simulink model "BMS_Submodel"  (R2026a)
settings: Solver=FixedStepAuto  StopTime=3600  FixedStep=0.01
values from neighbouring files (symbols this model uses):
  a_montes = 0.869    [WS_Variables.mat]
  alpha_cal = 0.384    [WS_Variables.mat]
  dt_h = 1    [WS_Variables.mat]    (also in validate_fixes.m)
  Ea_cal = 20592    [WS_Variables.mat]
  F_const = 96485    [WS_Variables.mat]
  I_ch_max = 3    [WS_Variables.mat]
  I_dis_max = 3    [WS_Variables.mat]
  k0_cal = 0.142    [WS_Variables.mat]
  kcal_ref = 0.0003694    [WS_Variables.mat]
  kCch = 0.1038    [WS_Variables.mat]
  kCdch = 0.296    [WS_Variables.mat]
  kcyc = 0.003414    [WS_Variables.mat]
  kDODc = 0.0046    [WS_Variables.mat]
  kmSOC = 0.0513    [WS_Variables.mat]
  kT = 5.8755    [WS_Variables.mat]
  mSOCref = 0.42    [WS_Variables.mat]
  Q_nom = 3    [WS_Variables.mat]
  R_ch_2D = [0.0536 0.0408 0.0368 0.0344 0.0288 0.0264 0.024 0.0595555555556 0.0453333333333 0.0408888888889 0.0382222222222 0.032 ... (77 elements, 7x11)]    [WS_Variables.mat]
  R_dis_2D = [0.1152 0.088 0.0768 0.072 0.064 0.0576 0.0528 0.0936 0.0715 0.0624 0.0585 0.052 ... (77 elements, 7x11)]    [WS_Variables.mat]
  R_gas = 8.314462618    [WS_Variables.mat]
  SOC0 = 0.5    [WS_Variables.mat]
  SOC_grid = [0 0.1 0.2 0.3 0.4 0.5 0.6 0.7 0.8 0.9 1]    [WS_Variables.mat]
  SOC_max = 0.95    [WS_Variables.mat]
  SOC_min = 0.05    [WS_Variables.mat]
  T_degC = 25    [WS_Variables.mat]
  T_grid_C = [10 20 25 30 40 50 60]    [WS_Variables.mat]
  Tref_cal = 298.15    [WS_Variables.mat]
  Tref_K = 298    [WS_Variables.mat]
  Ua_ref = 0.123    [WS_Variables.mat]
  V_nom = 3.2    [WS_Variables.mat]
undefined symbols (not defined in the file or in its folder): b_I, b_T, b_V, DiscIntNeverNeededParam, g_I, GridSearch_EN, I_cmd, nseedI, nseedT, nseedV, SOC0_est, SOH_Grid, step_size
libraries: simulink x5, sl_discontinuities x1
settings Model: Creator=diaag  LastModifiedBy=diaag

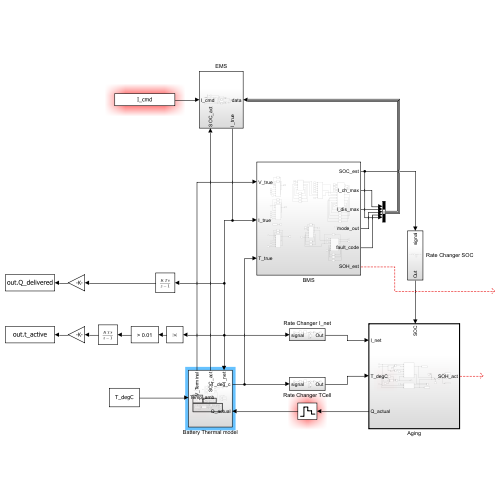
[thumbnail: Simulink's stored preview of the top-level diagram]
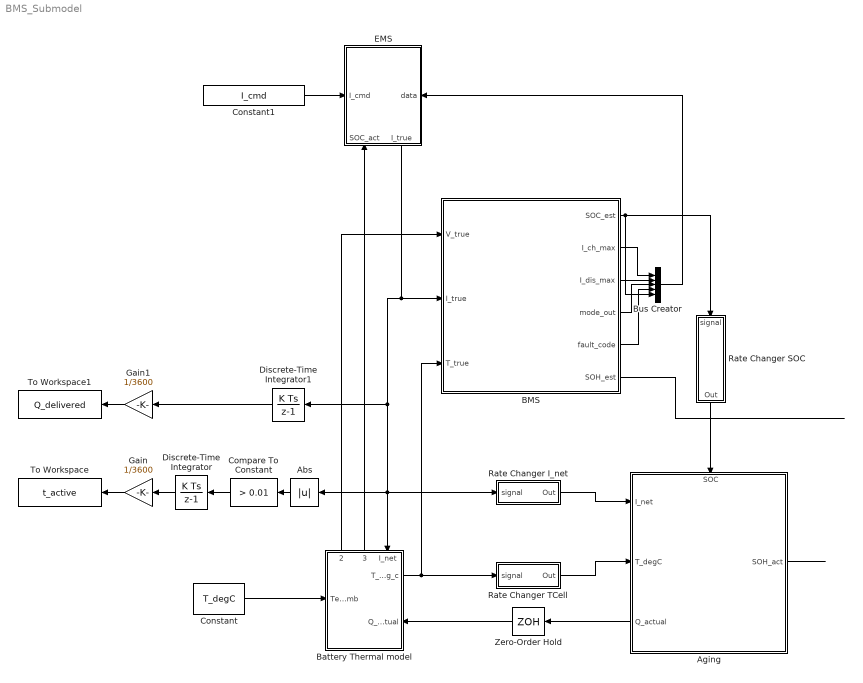
== system BMS_Submodel ==
  Abs : Abs  SaturateOnIntegerOverflow=off
  Aging : Subsystem  TreatAsAtomicUnit=on  SystemSampleTime=3600
      settings: PortSchema="{\"entries\":[{\"content\":{\"sides\":[{\"content\":{\"connectorIds\":[\"In1\",\"In2\",\"Out2\"]},\"type\":\"ConnectorPlacement.EquallySpacedRectSide\",\"uuid\":\"e6db651b-c6dd-4cac-b472-a1afbe19ba44\"},{\"content\":{\"connectorIds\":[\"Out1\"],\"side\":\"RIGHT\"},\"type\":\"ConnectorPlacement.EquallySpacedRectSide\",\"uuid\":\"7d47abdb-bdb7-40fd-84ce-b87800cb59fa\"},{\"content\":{\"connectorIds\":[\"In3\"],\"side\":\"TOP\"},\"type\":\"ConnectorPlacement.EquallySpacedRectSide\",\"uuid\":\"eff55775-1cf2-424a-af47-d3042302cf74\"}]},\"type\":\"ConnectorPlacement.EquallySpacedConnector\",\"uuid\":\"45aa8090-c1c1-4510-ac4d-5e24907f6a7b\"}],\"packageUris\":[\"http://schema.mathworks.com/mf0/Connector/R2020b\"],\"version\":\"1.0\"}"
  BMS : Subsystem
  Battery Thermal model : Subsystem
      settings: PortSchema="{\"entries\":[{\"content\":{\"sides\":[{\"content\":{\"connectorIds\":[\"Out2\",\"Out3\",\"In1\"]},\"type\":\"ConnectorPlacement.EquallySpacedRectSide\",\"uuid\":\"e701b896-6e4d-4329-a4c3-4a880497ce66\"},{\"content\":{\"side\":\"RIGHT\"},\"type\":\"ConnectorPlacement.EquallySpacedRectSide\",\"uuid\":\"c3e4b798-963d-4ee1-99ed-454cd6d82987\"},{\"content\":{\"connectorIds\":[\"In2\"],\"side\":\"TOP\"},\"type\":\"ConnectorPlacement.EquallySpacedRectSide\",\"uuid\":\"33ef008e-5290-4140-baf3-69d32b77873e\"},{\"content\":{\"connectorIds\":[\"Out1\",\"In3\"],\"side\":\"BOTTOM\"},\"type\":\"ConnectorPlacement.EquallySpacedRectSide\",\"uuid\":\"032c09d0-f76a-4e61-be97-2904950a15a3\"}]},\"type\":\"ConnectorPlacement.EquallySpacedConnector\",\"uuid\":\"523c5e39-84aa-4d7a-8c26-e0b756ae59f3\"}],\"packageUris\":[\"http://schema.mathworks.com/mf0/Connector/R2020b\"],\"version\":\"1.0\"}"
  Bus Creator : BusCreator  Inputs=5
  Compare To Constant : simulink/Logic and Bit Operations/Compare To Constant  relop=>  const=0.01  OutDataTypeStr=boolean
  Constant : Constant  Value=T_degC
  Constant1 : Constant  Value=I_cmd
  Discrete-Time Integrator : DiscreteIntegrator  SampleTime=-1  OutDataTypeStr=double  ICPrevOutput=DiscIntNeverNeededParam  ICPrevScaledInput=DiscIntNeverNeededParam
  Discrete-Time Integrator1 : DiscreteIntegrator  SampleTime=-1  ICPrevOutput=DiscIntNeverNeededParam  ICPrevScaledInput=DiscIntNeverNeededParam
  EMS : Subsystem
      settings: PortSchema="{\"entries\":[{\"content\":{\"sides\":[{\"content\":{\"connectorIds\":[\"In1\"]},\"type\":\"ConnectorPlacement.EquallySpacedRectSide\",\"uuid\":\"d23f0ade-e6c5-473f-be03-48db0421b0ac\"},{\"content\":{\"connectorIds\":[\"In3\"],\"side\":\"RIGHT\"},\"type\":\"ConnectorPlacement.EquallySpacedRectSide\",\"uuid\":\"35749c49-4500-4b94-810c-884c3143aa7f\"},{\"content\":{\"side\":\"TOP\"},\"type\":\"ConnectorPlacement.EquallySpacedRectSide\",\"uuid\":\"e0e4976e-0f30-4d6f-9552-049331019e02\"},{\"content\":{\"connectorIds\":[\"In2\",\"Out1\"],\"side\":\"BOTTOM\"},\"type\":\"ConnectorPlacement.EquallySpacedRectSide\",\"uuid\":\"1cb18c9d-5935-496e-9b55-fe9d42ae6b73\"}]},\"type\":\"ConnectorPlacement.EquallySpacedConnector\",\"uuid\":\"12474735-7fad-4afe-9583-bac38bcbc472\"}],\"packageUris\":[\"http://schema.mathworks.com/mf0/Connector/R2020b\"],\"version\":\"1.0\"}"
  Gain : Gain  Gain=1/3600  OutDataTypeStr=double
  Gain1 : Gain  Gain=1/3600  OutDataTypeStr=double
  Rate Changer I_net : Subsystem
  Rate Changer SOC : Subsystem
  Rate Changer TCell : Subsystem
  To Workspace : ToWorkspace  VariableName=t_active  SaveFormat=Timeseries  SampleTime=-1
      settings: MaxDataPoints=1
  To Workspace1 : ToWorkspace  VariableName=Q_delivered  SaveFormat=Timeseries  SampleTime=-1
      settings: MaxDataPoints=1
  Zero-Order Hold : ZeroOrderHold  SampleTime=3600/step_size
  wires:
  Rate Changer I_net/1(Out) -> Aging/1(I_net)
  Rate Changer SOC/1(Out) -> Aging/3(SOC)
  Rate Changer TCell/1(Out) -> Aging/2(T_degC)
  Zero-Order Hold/1 -> Battery Thermal model/3(Q_actual)
  Aging/2(Q_actual) -> Zero-Order Hold/1
  Battery Thermal model/1(T_deg_c) -> BMS/3(T_true), Rate Changer TCell/1(signal)
  Battery Thermal model/2(V_Terminal) -> BMS/1(V_true)
  EMS/1(I_true) -> Discrete-Time Integrator1/1, Abs/1, Rate Changer I_net/1(signal), Battery Thermal model/1(I_net), BMS/2(I_true)
  BMS/1(SOC_est) -> Rate Changer SOC/1(signal), Bus Creator/5
  BMS/6(SOH_est) -> ?
  Aging/1(SOH_act) -> ?
  BMS/2(I_ch_max) -> Bus Creator/1
  BMS/3(I_dis_max) -> Bus Creator/2
  BMS/4(mode_out) -> Bus Creator/3
  BMS/5(fault_code) -> Bus Creator/4
  Bus Creator/1 -> EMS/3(data)
  Constant/1 -> Battery Thermal model/2(Temp_amb)
  Constant1/1 -> EMS/1(I_cmd)
  Abs/1 -> Compare To Constant/1
  Compare To Constant/1 -> Discrete-Time Integrator/1
  Discrete-Time Integrator/1 -> Gain/1
  Gain/1 -> To Workspace/1
  Discrete-Time Integrator1/1 -> Gain1/1
  Gain1/1 -> To Workspace1/1
  Battery Thermal model/3(SOC_act) -> EMS/2(SOC_act)

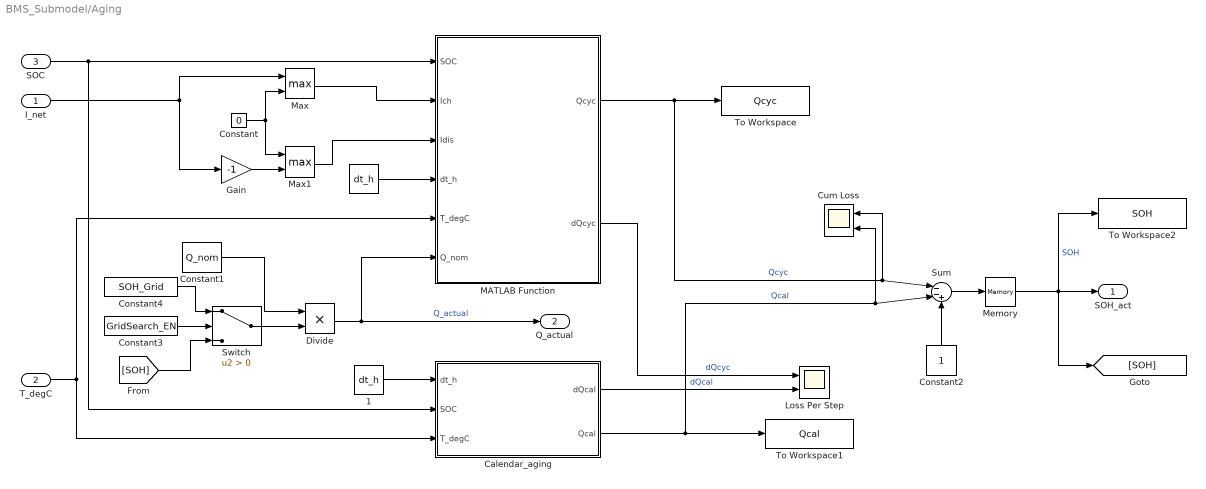
== system BMS_Submodel/Aging ==
  I_net : Inport
  T_degC : Inport  Port=2
  SOC : Inport  Port=3
  " " : Constant  Value=dt_h
  " 1" : Constant  Value=dt_h
  Calendar_aging : Subsystem
  Constant : Constant  Value=0
  Constant1 : Constant  Value=Q_nom
  Constant2 : Constant
  Constant3 : Constant  Value=GridSearch_EN
  Constant4 : Constant  Value=SOH_Grid
  Cum Loss : Scope  NumInputPorts=2
      settings: ActiveDisplayYMinimum=-1  ActiveDisplayYMaximum=1  DataLoggingVariableName=ScopeData5
  Divide : Product  Inputs=**
  Gain : Gain  Gain=-1
  Loss Per Step : Scope  NumInputPorts=2
      settings: ActiveDisplayYMinimum=-9E-6  ActiveDisplayYMaximum=2.1E-5
  MATLAB Function : MATLAB Function  TreatAsAtomicUnit=on
  Max : MinMax  Function=max  Inputs=2
  Max1 : MinMax  Function=max  Inputs=2
  Memory : Memory  InitialCondition=SOH_Grid  InheritSampleTime=on
  Sum : Sum  Inputs=|--+
  Switch : Switch  Criteria=u2 > Threshold  SaturateOnIntegerOverflow=off  InputSameDT=off
  To Workspace : ToWorkspace  VariableName=Qcyc  SaveFormat=Timeseries  SampleTime=-1
  To Workspace1 : ToWorkspace  VariableName=Qcal  SaveFormat=Timeseries  SampleTime=-1
  To Workspace2 : ToWorkspace  VariableName=SOH  SaveFormat=Timeseries  SampleTime=-1
  SOH_act : Outport
  Q_actual : Outport  Port=2
  wires:
  MATLAB Function/2(dQcyc) -> Loss Per Step/1  "dQcyc"
  T_degC/1 -> Calendar_aging/3(T_degC), MATLAB Function/5(T_degC)
  Calendar_aging/2(Qcal) -> To Workspace1/1, Sum/2, Cum Loss/2  "Qcal"
  Constant1/1 -> Divide/1
  Divide/1 -> MATLAB Function/6(Q_nom), Q_actual/1  "Q_actual"
  MATLAB Function/1(Qcyc) -> Sum/1, Cum Loss/1, To Workspace/1  "Qcyc"
  Calendar_aging/1(dQcal) -> Loss Per Step/2  "dQcal"
  Sum/1 -> Memory/1
  Memory/1 -> [SOH], To Workspace2/1, SOH_act/1  "SOH"
  Constant2/1 -> Sum/3
  SOC/1 -> MATLAB Function/1(SOC), Calendar_aging/2(SOC)
  " "/1 -> MATLAB Function/4(dt_h)
  " 1"/1 -> Calendar_aging/1(dt_h)
  I_net/1 -> Max/1, Gain/1
  Constant/1 -> Max/2, Max1/1
  Max1/1 -> MATLAB Function/3(Idis)
  Max/1 -> MATLAB Function/2(Ich)
  Gain/1 -> Max1/2
  Switch/1 -> Divide/2
  Constant4/1 -> Switch/1
  [SOH] -> Switch/3
  Constant3/1 -> Switch/2

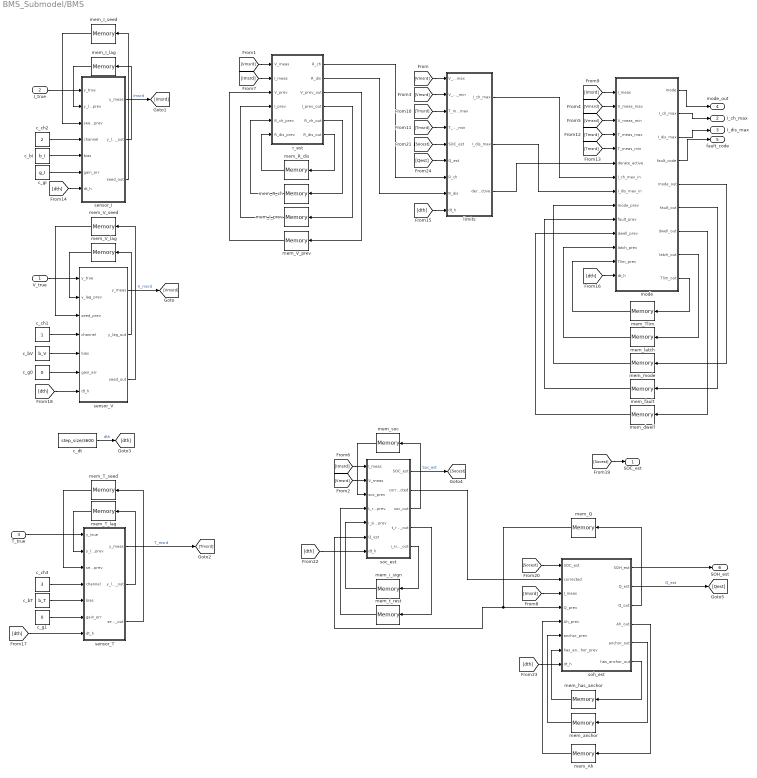
== system BMS_Submodel/BMS ==
  V_true : Inport
  I_true : Inport  Port=2
  T_true : Inport  Port=3
  c_bI : Constant  Value=b_I
  c_bT : Constant  Value=b_T
  c_bV : Constant  Value=b_V
  c_ch1 : Constant
  c_ch2 : Constant  Value=2
  c_ch3 : Constant  Value=3
  c_dt : Constant  Value=step_size/3600
  c_g0 : Constant  Value=0
  c_g1 : Constant  Value=0
  c_gI : Constant  Value=g_I
  limits : MATLAB Function  TreatAsAtomicUnit=on
  mem_Ah : Memory
  mem_I_lag : Memory
  mem_I_prev : Memory
  mem_I_seed : Memory  InitialCondition=nseedI
  mem_Q : Memory  InitialCondition=3.0
  mem_R_ch : Memory  InitialCondition=0.043
  mem_R_dis : Memory  InitialCondition=0.050
  mem_T_lag : Memory
  mem_T_seed : Memory  InitialCondition=nseedT
  mem_Tlim : Memory
  mem_V_lag : Memory
  mem_V_prev : Memory  InitialCondition=3.28
  mem_V_seed : Memory  InitialCondition=nseedV
  mem_anchor : Memory
  mem_dwell : Memory
  mem_fault : Memory
  mem_has_anchor : Memory
  mem_i_sign : Memory
  mem_latch : Memory
  mem_mode : Memory
  mem_soc : Memory  InitialCondition=SOC0_est
  mem_t_rest : Memory
  mode : MATLAB Function  TreatAsAtomicUnit=on
  r_est : MATLAB Function  TreatAsAtomicUnit=on
  sensor_I : MATLAB Function  TreatAsAtomicUnit=on
  sensor_T : MATLAB Function  TreatAsAtomicUnit=on
  sensor_V : MATLAB Function  TreatAsAtomicUnit=on
  soc_est : MATLAB Function  TreatAsAtomicUnit=on
  soh_est : MATLAB Function  TreatAsAtomicUnit=on
  SOC_est : Outport
  I_ch_max : Outport  Port=2
  I_dis_max : Outport  Port=3
  mode_out : Outport  Port=4
  fault_code : Outport  Port=5
  SOH_est : Outport  Port=6
  wires:
  r_est/3(V_prev_out) -> mem_V_prev/1
  soh_est/3(Q_out) -> mem_Q/1
  r_est/2(R_dis) -> limits/8(R_dis)
  soh_est/4(Ah_out) -> mem_Ah/1
  soh_est/5(anchor_out) -> mem_anchor/1
  soh_est/6(has_anchor_out) -> mem_has_anchor/1
  mem_i_sign/1 -> soc_est/5(i_sign_prev)
  mem_Q/1 -> soh_est/4(Q_prev), soc_est/6(Q_est)
  soc_est/5(i_sign_out) -> mem_i_sign/1
  mem_Ah/1 -> soh_est/5(Ah_prev)
  mem_anchor/1 -> soh_est/6(anchor_prev)
  mem_has_anchor/1 -> soh_est/7(has_anchor_prev)
  mode/1(mode) -> mode_out/1
  mem_I_prev/1 -> r_est/4(I_prev)
  soc_est/2(corrected) -> soh_est/2(corrected)
  mem_R_dis/1 -> r_est/6(R_dis_prev)
  mem_R_ch/1 -> r_est/5(R_ch_prev)
  soc_est/3(soc_out) -> mem_soc/1
  mem_soc/1 -> soc_est/3(soc_prev)
  soc_est/4(t_rest_out) -> mem_t_rest/1
  mem_t_rest/1 -> soc_est/4(t_rest_prev)
  r_est/1(R_ch) -> limits/7(R_ch)
  limits/2(I_dis_max) -> mode/8(I_dis_max_in)
  r_est/4(I_prev_out) -> mem_I_prev/1
  r_est/5(R_ch_out) -> mem_R_ch/1
  r_est/6(R_dis_out) -> mem_R_dis/1
  mem_V_prev/1 -> r_est/3(V_prev)
  limits/1(I_ch_max) -> mode/7(I_ch_max_in)
  limits/3(derate_active) -> mode/6(derate_active)
  mode/2(I_ch_max) -> I_ch_max/1
  mode/3(I_dis_max) -> I_dis_max/1
  mode/4(fault_code) -> fault_code/1
  mode/5(mode_out) -> mem_mode/1
  mode/6(fault_out) -> mem_fault/1
  mode/7(dwell_out) -> mem_dwell/1
  mode/8(latch_out) -> mem_latch/1
  mode/9(Tlim_out) -> mem_Tlim/1
  mem_dwell/1 -> mode/11(dwell_prev)
  mem_fault/1 -> mode/10(fault_prev)
  mem_mode/1 -> mode/9(mode_prev)
  mem_latch/1 -> mode/12(latch_prev)
  mem_Tlim/1 -> mode/13(Tlim_prev)
  [Vmsrd] -> limits/1(V_meas_max)
  [Vmsrd] -> r_est/1(V_meas)
  [Vmsrd] -> soc_est/2(V_meas)
  [Vmsrd] -> limits/2(V_meas_min)
  [Vmsrd] -> mode/2(V_meas_max)
  [Vmsrd] -> mode/3(V_meas_min)
  [Imsrd] -> soc_est/1(I_meas)
  [Imsrd] -> r_est/2(I_meas)
  [Imsrd] -> soh_est/3(I_meas)
  [Imsrd] -> mode/1(I_meas)
  [Tmsrd] -> limits/3(T_meas_max)
  [Tmsrd] -> limits/4(T_meas_min)
  [Tmsrd] -> mode/4(T_meas_max)
  [Tmsrd] -> mode/5(T_meas_min)
  [dth] -> limits/9(dt_h)
  [dth] -> mode/14(dt_h)
  soc_est/1(SOC_est) -> [Socest]  "Soc_est"
  [Socest] -> SOC_est/1
  [Socest] -> soh_est/1(SOC_est)
  [Socest] -> limits/5(SOC_est)
  soh_est/1(SOH_est) -> SOH_est/1
  sensor_V/3(seed_out) -> mem_V_seed/1
  mem_I_lag/1 -> sensor_I/2(y_lag_prev)
  mem_I_seed/1 -> sensor_I/3(seed_prev)
  I_true/1 -> sensor_I/1(y_true)
  V_true/1 -> sensor_V/1(y_true)
  c_bI/1 -> sensor_I/5(bias)
  sensor_T/3(seed_out) -> mem_T_seed/1
  c_ch2/1 -> sensor_I/4(channel)
  c_gI/1 -> sensor_I/6(gain_err)
  sensor_I/3(seed_out) -> mem_I_seed/1
  c_ch3/1 -> sensor_T/4(channel)
  sensor_I/1(y_meas) -> [Imsrd]  "Imsrd"
  sensor_V/2(y_lag_out) -> mem_V_lag/1
  sensor_T/1(y_meas) -> [Tmsrd]  "T_msrd"
  c_bT/1 -> sensor_T/5(bias)
  c_g0/1 -> sensor_V/6(gain_err)
  mem_T_seed/1 -> sensor_T/3(seed_prev)
  mem_T_lag/1 -> sensor_T/2(y_lag_prev)
  sensor_V/1(y_meas) -> [Vmsrd]  "V_msrd"
  mem_V_lag/1 -> sensor_V/2(y_lag_prev)
  mem_V_seed/1 -> sensor_V/3(seed_prev)
  [dth] -> sensor_V/7(dt_h)
  sensor_I/2(y_lag_out) -> mem_I_lag/1
  sensor_T/2(y_lag_out) -> mem_T_lag/1
  [dth] -> sensor_I/7(dt_h)
  c_bV/1 -> sensor_V/5(bias)
  T_true/1 -> sensor_T/1(y_true)
  c_ch1/1 -> sensor_V/4(channel)
  [dth] -> sensor_T/7(dt_h)
  c_dt/1 -> [dth]  "dth"
  [dth] -> soc_est/7(dt_h)
  [dth] -> soh_est/8(dt_h)
  soh_est/2(Q_est) -> [Qest]  "Q_est"
  [Qest] -> limits/6(Q_est)
  c_g1/1 -> sensor_T/6(gain_err)

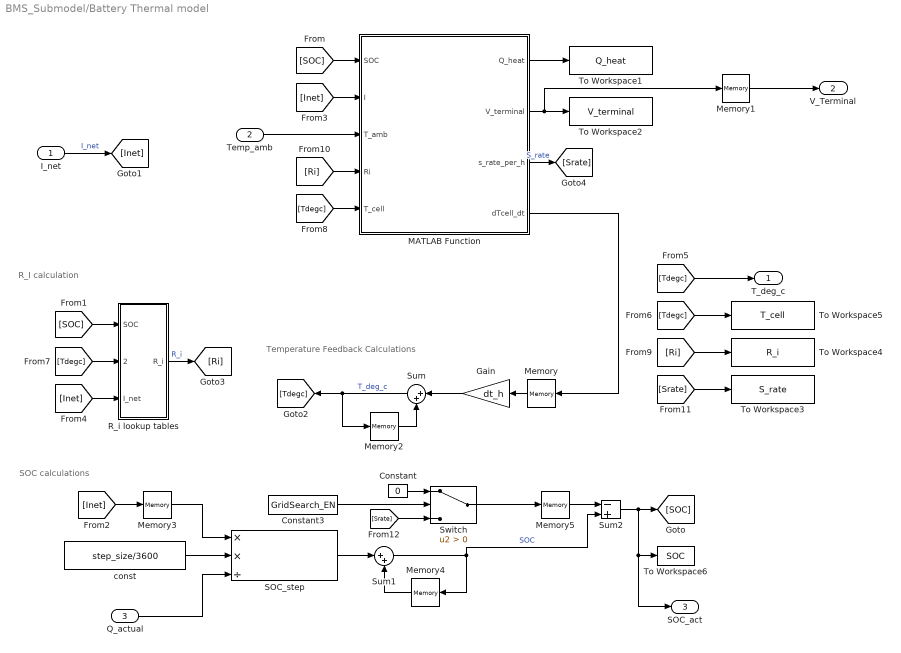
== system BMS_Submodel/Battery Thermal model ==
  note: Temperature Feedback Calculations
  note: SOC calculations
  note: R_I calculation
  I_net : Inport
  Temp_amb : Inport  Port=2
  Q_actual : Inport  Port=3
  Constant : Constant  Value=0
  Constant3 : Constant  Value=GridSearch_EN
  Gain : Gain  Gain=dt_h
  MATLAB Function : MATLAB Function  TreatAsAtomicUnit=on
  Memory : Memory
  Memory1 : Memory  InitialCondition=V_nom
  Memory2 : Memory  InitialCondition=T_degC
  Memory3 : Memory
  Memory4 : Memory  InitialCondition=SOC0
  Memory5 : Memory
  R_i lookup tables : Subsystem
  SOC_step : Product  Inputs=**/
  Sum : Sum  Inputs=|++
  Sum1 : Sum  Inputs=|++
  Sum2 : Sum  Inputs=-+
  Switch : Switch  Criteria=u2 > Threshold  SaturateOnIntegerOverflow=off  InputSameDT=off
  To Workspace1 : ToWorkspace  VariableName=Q_heat  SaveFormat=Timeseries  SampleTime=-1
  To Workspace2 : ToWorkspace  VariableName=V_terminal  SaveFormat=Timeseries  SampleTime=-1
  To Workspace3 : ToWorkspace  VariableName=S_rate  SaveFormat=Timeseries  SampleTime=-1
  To Workspace4 : ToWorkspace  VariableName=R_i  SaveFormat=Timeseries  SampleTime=-1
  To Workspace5 : ToWorkspace  VariableName=T_cell  SaveFormat=Timeseries  SampleTime=-1
  To Workspace6 : ToWorkspace  VariableName=SOC  SaveFormat=Timeseries  SampleTime=-1
      settings: MaxDataPoints=1
  const : Constant  Value=step_size/3600
  T_deg_c : Outport
  V_Terminal : Outport  Port=2
  SOC_act : Outport  Port=3
  wires:
  MATLAB Function/1(Q_heat) -> To Workspace1/1
  [SOC] -> MATLAB Function/1(SOC)
  Temp_amb/1 -> MATLAB Function/3(T_amb)
  MATLAB Function/2(V_terminal) -> To Workspace2/1, Memory1/1
  MATLAB Function/4(dTcell_dt) -> Memory/1
  Memory/1 -> Gain/1
  Sum/1 -> [Tdegc], Memory2/1  "T_deg_c"
  Gain/1 -> Sum/1
  Memory2/1 -> Sum/2
  Memory1/1 -> V_Terminal/1
  SOC_step/1 -> Sum1/1
  Memory4/1 -> Sum1/2
  Memory3/1 -> SOC_step/1
  const/1 -> SOC_step/2
  Sum1/1 -> Sum2/2, Memory4/1  "SOC"
  Sum2/1 -> SOC_act/1, To Workspace6/1, [SOC]
  [SOC] -> R_i lookup tables/1(SOC)
  Q_actual/1 -> SOC_step/3
  I_net/1 -> [Inet]  "I_net"
  [Inet] -> Memory3/1
  [Inet] -> MATLAB Function/2(I)
  [Inet] -> R_i lookup tables/3(I_net)
  [Tdegc] -> T_deg_c/1
  [Tdegc] -> To Workspace5/1
  [Tdegc] -> R_i lookup tables/2(T_cell)
  [Tdegc] -> MATLAB Function/5(T_cell)
  R_i lookup tables/1(R_i) -> [Ri]  "R_i"
  [Ri] -> To Workspace4/1
  [Ri] -> MATLAB Function/4(Ri)
  Memory5/1 -> Sum2/1
  MATLAB Function/3(s_rate_per_h) -> [Srate]  "S_rate"
  [Srate] -> To Workspace3/1
  Switch/1 -> Memory5/1
  Constant3/1 -> Switch/2
  [Srate] -> Switch/3
  Constant/1 -> Switch/1

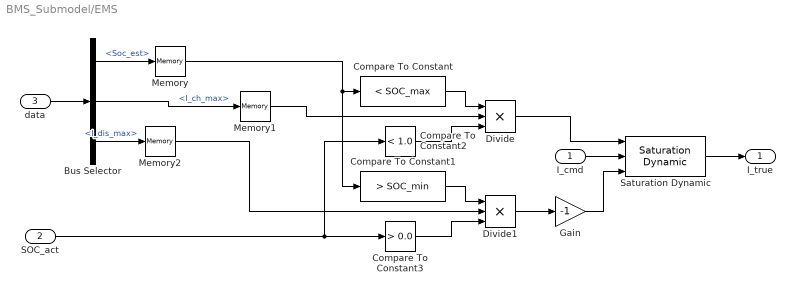
== system BMS_Submodel/EMS ==
  I_cmd : Inport
  SOC_act : Inport  Port=2
  data : Inport  Port=3
  Bus Selector : BusSelector  OutputSignals=Soc_est,I_ch_max,I_dis_max
  Compare To Constant : simulink/Logic and Bit Operations/Compare To Constant  relop=<  const=SOC_max  OutDataTypeStr=boolean
  Compare To Constant1 : simulink/Logic and Bit Operations/Compare To Constant  relop=>  const=SOC_min  OutDataTypeStr=boolean
  Compare To Constant2 : simulink/Logic and Bit Operations/Compare To Constant  relop=<  const=1.0  OutDataTypeStr=uint8
  Compare To Constant3 : simulink/Logic and Bit Operations/Compare To Constant  relop=>  const=0.0  OutDataTypeStr=uint8
  Divide : Product  Inputs=***  OutDataTypeStr=double
  Divide1 : Product  Inputs=***  OutDataTypeStr=double
  Gain : Gain  Gain=-1
  Memory : Memory  InitialCondition=SOC0
  Memory1 : Memory  InitialCondition=I_ch_max
  Memory2 : Memory  InitialCondition=I_dis_max
  Saturation Dynamic : sl_discontinuities/Saturation Dynamic  OutMin=[]  OutMax=[]  OutDataTypeStr=Inherit: Same as second input  OutDataType=fixdt(1, 16)  OutScaling=2^-10  DoSatur=off
      settings: LibrarySourceBlock=|
      | simulink/Discontinuities/Saturation
      | Dynamic
  I_true : Outport
  wires:
  Memory1/1 -> Divide/2
  Saturation Dynamic/1 -> I_true/1
  Bus Selector/2 -> Memory1/1  "<I_ch_max>"
  data/1 -> Bus Selector/1
  Divide/1 -> Saturation Dynamic/1
  Memory2/1 -> Divide1/2
  Memory/1 -> Compare To Constant1/1, Compare To Constant/1
  Bus Selector/3 -> Memory2/1  "<I_dis_max>"
  Divide1/1 -> Gain/1
  Bus Selector/1 -> Memory/1  "<Soc_est>"
  SOC_act/1 -> Compare To Constant3/1, Compare To Constant2/1
  Compare To Constant/1 -> Divide/1
  Compare To Constant2/1 -> Divide/3
  Compare To Constant1/1 -> Divide1/1
  Compare To Constant3/1 -> Divide1/3
  I_cmd/1 -> Saturation Dynamic/2
  Gain/1 -> Saturation Dynamic/3

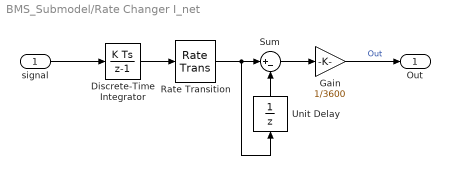
== system BMS_Submodel/Rate Changer I_net ==
  signal : Inport
  Discrete-Time Integrator : DiscreteIntegrator  SampleTime=-1  ICPrevOutput=DiscIntNeverNeededParam  ICPrevScaledInput=DiscIntNeverNeededParam
  Gain : Gain  Gain=1/3600
  Rate Transition : RateTransition  OutPortSampleTime=3600
  Sum : Sum  Inputs=|+-
  Unit Delay : UnitDelay  SampleTime=3600
  Out : Outport
  wires:
  Discrete-Time Integrator/1 -> Rate Transition/1
  Rate Transition/1 -> Unit Delay/1, Sum/1
  Gain/1 -> Out/1  "Out"
  signal/1 -> Discrete-Time Integrator/1
  Unit Delay/1 -> Sum/2
  Sum/1 -> Gain/1

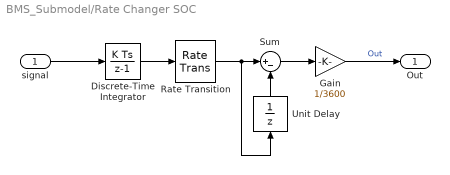
== system BMS_Submodel/Rate Changer SOC ==
  signal : Inport
  Discrete-Time Integrator : DiscreteIntegrator  SampleTime=-1  ICPrevOutput=DiscIntNeverNeededParam  ICPrevScaledInput=DiscIntNeverNeededParam
  Gain : Gain  Gain=1/3600
  Rate Transition : RateTransition  OutPortSampleTime=3600
  Sum : Sum  Inputs=|+-
  Unit Delay : UnitDelay  SampleTime=3600
  Out : Outport
  wires:
  Discrete-Time Integrator/1 -> Rate Transition/1
  Rate Transition/1 -> Unit Delay/1, Sum/1
  Gain/1 -> Out/1  "Out"
  signal/1 -> Discrete-Time Integrator/1
  Unit Delay/1 -> Sum/2
  Sum/1 -> Gain/1

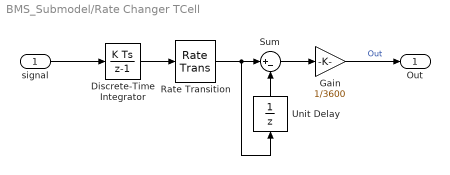
== system BMS_Submodel/Rate Changer TCell ==
  signal : Inport
  Discrete-Time Integrator : DiscreteIntegrator  SampleTime=-1  ICPrevOutput=DiscIntNeverNeededParam  ICPrevScaledInput=DiscIntNeverNeededParam
  Gain : Gain  Gain=1/3600
  Rate Transition : RateTransition  OutPortSampleTime=3600
  Sum : Sum  Inputs=|+-
  Unit Delay : UnitDelay  SampleTime=3600
  Out : Outport
  wires:
  Discrete-Time Integrator/1 -> Rate Transition/1
  Rate Transition/1 -> Unit Delay/1, Sum/1
  Gain/1 -> Out/1  "Out"
  signal/1 -> Discrete-Time Integrator/1
  Unit Delay/1 -> Sum/2
  Sum/1 -> Gain/1

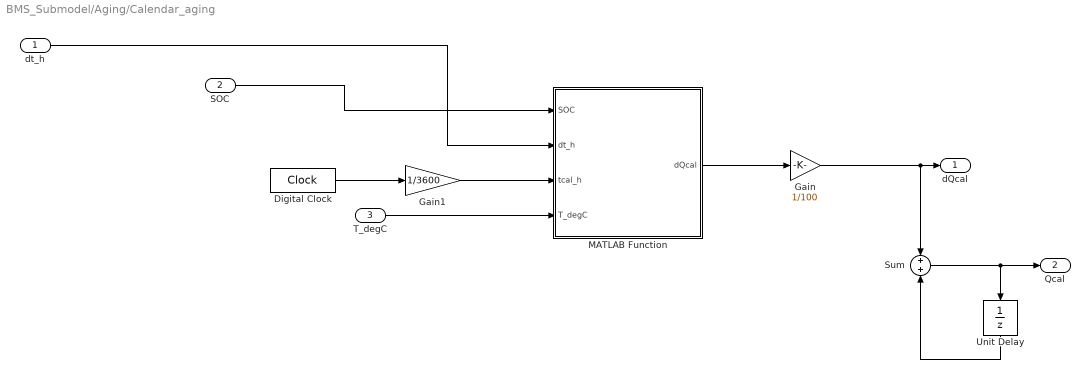
== system BMS_Submodel/Aging/Calendar_aging ==
  dt_h : Inport
  SOC : Inport  Port=2
  T_degC : Inport  Port=3
  Digital Clock : DigitalClock  SampleTime=3600
  Gain : Gain  Gain=1/100
  Gain1 : Gain  Gain=1/3600
  MATLAB Function : MATLAB Function  TreatAsAtomicUnit=on
  Sum : Sum
  Unit Delay : UnitDelay  SampleTime=3600
  dQcal : Outport
  Qcal : Outport  Port=2
  wires:
  SOC/1 -> MATLAB Function/1(SOC)
  Digital Clock/1 -> Gain1/1
  dt_h/1 -> MATLAB Function/2(dt_h)
  MATLAB Function/1(dQcal) -> Gain/1
  T_degC/1 -> MATLAB Function/4(T_degC)
  Gain/1 -> Sum/1, dQcal/1
  Sum/1 -> Unit Delay/1, Qcal/1
  Gain1/1 -> MATLAB Function/3(tcal_h)
  Unit Delay/1 -> Sum/2

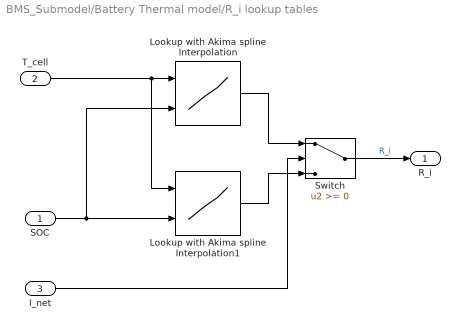
== system BMS_Submodel/Battery Thermal model/R_i lookup tables ==
  SOC : Inport
  T_cell : Inport  Port=2
  I_net : Inport  Port=3
  Lookup with Akima spline Interpolation : Lookup_n-D  BreakpointsForDimension1=T_grid_C  BreakpointsForDimension2=SOC_grid  Table=R_ch_2D  InterpMethod=Akima spline  InternalRulePriority=Speed  RndMeth=Simplest
      settings: InputPortMap=u0,u1
  Lookup with Akima spline Interpolation1 : Lookup_n-D  BreakpointsForDimension1=T_grid_C  BreakpointsForDimension2=SOC_grid  Table=R_dis_2D  InterpMethod=Akima spline  InternalRulePriority=Speed  RndMeth=Simplest
      settings: InputPortMap=u0,u1
  Switch : Switch  SaturateOnIntegerOverflow=off  InputSameDT=off
  R_i : Outport
  wires:
  Lookup with Akima spline Interpolation/1 -> Switch/1
  Switch/1 -> R_i/1  "R_i"
  SOC/1 -> Lookup with Akima spline Interpolation/2, Lookup with Akima spline Interpolation1/2
  Lookup with Akima spline Interpolation1/1 -> Switch/3
  I_net/1 -> Switch/2
  T_cell/1 -> Lookup with Akima spline Interpolation1/1, Lookup with Akima spline Interpolation/1

== matlab function BMS_Submodel/BMS/sensor_T ==
  data: y_true input; y_meas output; y_lag_prev input; seed_prev input; channel input; bias input; gain_err input; dt_h input; y_lag_out output; seed_out output
function [y_meas, y_lag_out, seed_out] = sensor_T(y_true, y_lag_prev, seed_prev, channel, bias, gain_err, dt_h)
[y_meas, y_lag_out, seed_out] = bms_sensor_model_sl(y_true, y_lag_prev, seed_prev, channel, bias, gain_err, dt_h);
end

== matlab function BMS_Submodel/BMS/r_est ==
  data: V_meas input; R_ch output; I_meas input; V_prev input; I_prev input; R_ch_prev input; R_dis_prev input; R_dis output; V_prev_out output; I_prev_out output; R_ch_out output; R_dis_out output
function [R_ch, R_dis, V_prev_out, I_prev_out, R_ch_out, R_dis_out] = r_est(V_meas, I_meas, V_prev, I_prev, R_ch_prev, R_dis_prev)
[R_ch, R_dis, V_prev_out, I_prev_out, R_ch_out, R_dis_out] = bms_r_estimator_sl(V_meas, I_meas, V_prev, I_prev, R_ch_prev, R_dis_prev);
end

== matlab function BMS_Submodel/BMS/soc_est ==
  data: I_meas input; SOC_est output; V_meas input; soc_prev input; t_rest_prev input; i_sign_prev input; Q_est input; dt_h input; corrected output; soc_out output; t_rest_out output; i_sign_out output
function [SOC_est, corrected, soc_out, t_rest_out, i_sign_out] = soc_est(I_meas, V_meas, soc_prev, t_rest_prev, i_sign_prev, Q_est, dt_h)
[SOC_est, corrected, soc_out, t_rest_out, i_sign_out] = bms_soc_estimator_sl(I_meas, V_meas, soc_prev, t_rest_prev, i_sign_prev, Q_est, dt_h);
end

== matlab function BMS_Submodel/BMS/soh_est ==
  data: SOC_est input; SOH_est output; corrected input; I_meas input; Q_prev input; Ah_prev input; anchor_prev input; has_anchor_prev input; dt_h input; Q_est output; Q_out output; Ah_out output; anchor_out output; has_anchor_out output
function [SOH_est, Q_est, Q_out, Ah_out, anchor_out, has_anchor_out] = soh_est(SOC_est, corrected, I_meas, Q_prev, Ah_prev, anchor_prev, has_anchor_prev, dt_h)
[SOH_est, Q_est, Q_out, Ah_out, anchor_out, has_anchor_out] = bms_soh_estimator_sl(SOC_est, corrected, I_meas, Q_prev, Ah_prev, anchor_prev, has_anchor_prev, dt_h);
end

== matlab function BMS_Submodel/BMS/limits ==
  data: V_meas_max input; I_ch_max output; V_meas_min input; T_meas_max input; T_meas_min input; SOC_est input; Q_est input; R_ch input; R_dis input; dt_h input; I_dis_max output; derate_active output
function [I_ch_max, I_dis_max, derate_active] = limits(V_meas_max, V_meas_min, T_meas_max, T_meas_min, SOC_est, Q_est, R_ch, R_dis, dt_h)
[I_ch_max, I_dis_max, derate_active] = bms_limits_sl(V_meas_max, V_meas_min, T_meas_max, T_meas_min, SOC_est, Q_est, R_ch, R_dis, dt_h);
end

== matlab function BMS_Submodel/BMS/mode ==
  data: I_meas input; mode output; V_meas_max input; V_meas_min input; T_meas_max input; T_meas_min input; derate_active input; I_ch_max_in input; I_dis_max_in input; mode_prev input; fault_prev input; dwell_prev input; latch_prev input; Tlim_prev input; dt_h input; I_ch_max output; I_dis_max output; fault_code output; mode_out output; fault_out output; dwell_out output; latch_out output; Tlim_out output
function [ mode, I_ch_max, I_dis_max, fault_code, mode_out, fault_out, dwell_out, latch_out, Tlim_out] = mode( I_meas, V_meas_max, V_meas_min, T_meas_max, T_meas_min, derate_active, I_ch_max_in, I_dis_max_in, mode_prev, fault_prev, dwell_prev, latch_prev, Tlim_prev, dt_h)
[mode, I_ch_max, I_dis_max, fault_code, mode_out, fault_out, dwell_out, latch_out, Tlim_out] = bms_mode_sl(I_meas, V_meas_max, V_meas_min, T_meas_max, T_meas_min, derate_active, I_ch_max_in, I_dis_max_in, mode_prev, fault_prev, dwell_prev, latch_prev, Tlim_prev, dt_h);
end

== matlab function BMS_Submodel/Aging/Calendar_aging/MATLAB Function ==
  data: SOC input; dQcal output; dt_h input; tcal_h input; T_degC input; Ea_cal parameter; R_gas parameter; Tref_cal parameter; alpha_cal parameter; F_const parameter; Ua_ref parameter; k0_cal parameter; kcal_ref parameter
function dQcal = calendar_aging(SOC, dt_h, tcal_h, T_degC, ...
    Ea_cal, R_gas, Tref_cal, alpha_cal, F_const, Ua_ref, k0_cal, kcal_ref)

dQcal = calendar_aging(SOC, dt_h, tcal_h, T_degC, ...
    Ea_cal, R_gas, Tref_cal, alpha_cal, F_const, Ua_ref, k0_cal, kcal_ref);
end

== matlab function BMS_Submodel/BMS/sensor_V ==
  data: y_true input; y_meas output; y_lag_prev input; seed_prev input; channel input; bias input; gain_err input; dt_h input; y_lag_out output; seed_out output
function [y_meas, y_lag_out, seed_out] = sensor_V(y_true, y_lag_prev, seed_prev, channel, bias, gain_err, dt_h)
[y_meas, y_lag_out, seed_out] = bms_sensor_model_sl(y_true, y_lag_prev, seed_prev, channel, bias, gain_err, dt_h);
end

== matlab function BMS_Submodel/Aging/MATLAB Function ==
  settings: updateMethod=DISCRETE
  data: SOC input; Qcyc output; Ich input; Idis input; dt_h input; T_degC input; Q_nom input; kT parameter; Tref_K parameter; kDODc parameter; kcyc parameter; kCch parameter; kCdch parameter; kmSOC parameter; mSOCref parameter; a_montes parameter; dQcyc output
function [Qcyc, dQcyc] = cycle_aging(SOC, Ich, Idis, dt_h, T_degC, Q_nom, ...
    kT, Tref_K, kDODc, kcyc, kCch, kCdch, kmSOC, mSOCref, a_montes)

[Qcyc, dQcyc] = cycle_aging(SOC, Ich, Idis, dt_h, T_degC, Q_nom, ...
    kT, Tref_K, kDODc, kcyc, kCch, kCdch, kmSOC, mSOCref, a_montes);

Qcyc = Qcyc / 100;
dQcyc = dQcyc / 100;

end

== matlab function BMS_Submodel/Battery Thermal model/MATLAB Function ==
  data: SOC input; I input; T_amb input; Q_heat output; V_terminal output; s_rate_per_h output; dTcell_dt output; Ri input; T_cell input
function [Q_heat, V_terminal, s_rate_per_h, dTcell_dt] = cell_thermal(SOC, I,T_amb,Ri, T_cell)

  [Q_heat, V_terminal, s_rate_per_h, dTcell_dt] = cell_thermal(SOC, I,T_cell, T_amb,Ri);

end

== matlab function BMS_Submodel/BMS/sensor_I ==
  data: y_true input; y_meas output; y_lag_prev input; seed_prev input; channel input; bias input; gain_err input; dt_h input; y_lag_out output; seed_out output
function [y_meas, y_lag_out, seed_out] = sensor_I(y_true, y_lag_prev, seed_prev, channel, bias, gain_err, dt_h)
[y_meas, y_lag_out, seed_out] = bms_sensor_model_sl(y_true, y_lag_prev, seed_prev, channel, bias, gain_err, dt_h);
end
